simulink model "engine_with_transmission"  (R2026a)
settings: Solver=VariableStepAuto  StopTime=10
libraries: fl_lib x45, nesl_utility x29, sdl_lib x14
settings Model: Creator=doyeop  LastModifiedBy=doyeop

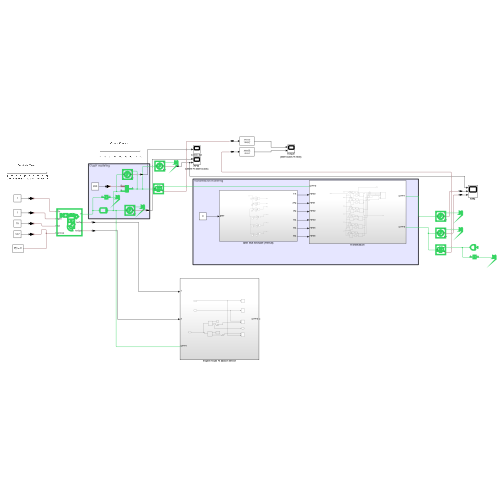
[thumbnail: Simulink's stored preview of the top-level diagram]
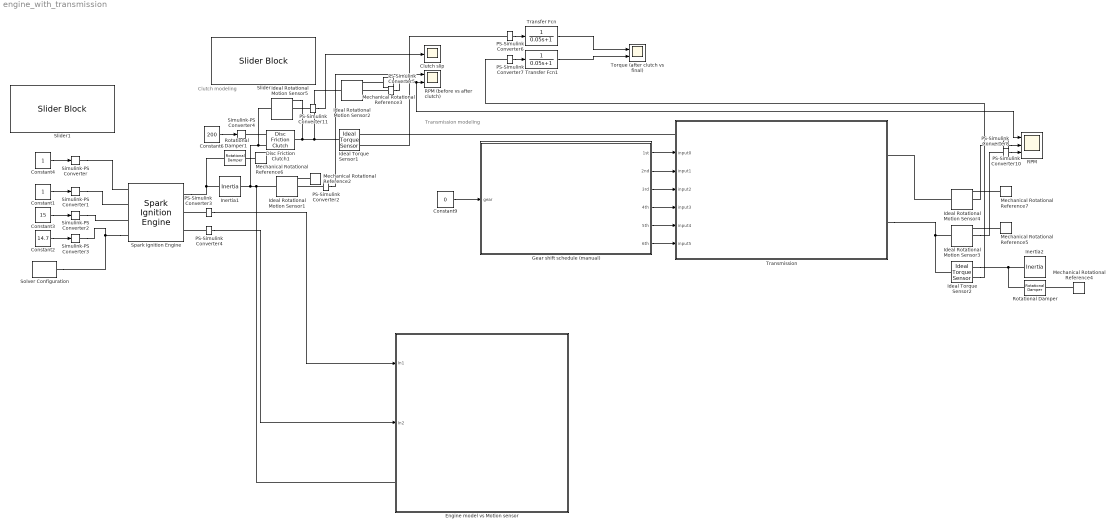
== system engine_with_transmission ==
  note: Transmission modeling
  note: Clutch modeling
  Clutch slip : Scope
      settings: ActiveDisplayYMinimum=-1  ActiveDisplayYMaximum=1  DataLoggingVariableName=ScopeData8
  Constant1 : Constant
  Constant2 : Constant  Value=14.7  SampleTime=-1
  Constant3 : Constant  Value=15  SampleTime=-1
  Constant4 : Constant  SampleTime=-1
  Constant6 : Constant  Value=200  SampleTime=-1
  Constant9 : Constant  Value=0
  Disc Friction Clutch1 : sdl_lib/Clutches/Disc Friction Clutch  geometry_model=sdl.enum.friction_geometry.radius  r_eff=130 mm  d_o=150 mm  d_i=100 mm  nS=4  piston_area=0.001 m^2  unidirectional=sdl.enum.directionality.bidirectional  friction_model=sdl.enum.friction_model_TLU_thermal.fixed  mu_w_vector=[0, 100, 1000] rad/s  temperature_TLU=[280, 300, 320] K  mu_static=0.35  mu_static_vector=[.4, .38, .36]  mu_coulomb=0.3  mu_coulomb_vector=[.3, .22, .19]  mu_coulomb_temp_vector=[.3, .28, .25]  mu_coulomb_matrix=[.34, .32, .3; .3, .28, .25; .25, .2, .15]  mu_interp_method=simscape.enum.interpolation.linear  mu_extrap_method=simscape.enum.extrapolation.linear  d_f=1  w_tol=0.001 rad/s  pressure_min=100 Pa  mu_visc=0 N*m*s/rad  initial_state_locked=sdl.enum.initial_lock.unlocked  thermal_mass=50 kJ/K  T_init=300 K
  Engine model vs Motion sensor : Subsystem
  Gear shift schedule (manual) : Subsystem
  Ideal Rotational Motion Sensor{1..5} (5 alike) : fl_lib/Mechanical/Mechanical Sensors/Ideal Rotational Motion Sensor  reference=foundation.enum.MeasurementReference.difference  acceleration_port=false  velocity_port=true  position_port=true  wrap_angle=false  offset=0 rad
  Ideal Torque Sensor1 : fl_lib/Mechanical/Mechanical Sensors/Ideal Torque Sensor
  Ideal Torque Sensor2 : fl_lib/Mechanical/Mechanical Sensors/Ideal Torque Sensor
  Inertia1 : fl_lib/Mechanical/Rotational Elements/Inertia  inertia=0.01 kg*m^2  num_ports=foundation.enum.numPorts2.two  w_specify=on  w_priority=Low  w=800 rpm  w_nominal_specify=off  w_nominal_value=1  w_nominal_unit=rad/s  t_specify=off  t_priority=None  t=0 N*m  t_nominal_specify=off  t_nominal_value=1  t_nominal_unit=N*m
  Inertia2 : fl_lib/Mechanical/Rotational Elements/Inertia  inertia=0.05 kg*m^2  num_ports=foundation.enum.numPorts2.one  w_specify=on  w_priority=None  w=0 rpm  w_nominal_specify=off  w_nominal_value=1  w_nominal_unit=rad/s  t_specify=off  t_priority=None  t=0 N*m  t_nominal_specify=off  t_nominal_value=1  t_nominal_unit=N*m
  Mechanical Rotational Reference{2..7} (6 alike) : fl_lib/Mechanical/Rotational Elements/Mechanical Rotational Reference
  PS-Simulink Converter{2,4..5,8,10..11} (6 alike) : nesl_utility/PS-Simulink Converter  PhysicalDomain=network_engine_domain  SubClassName=ps_output  LeftPortType=input  RightPortType=output  PseudoPeriodic=off  Frequencies=[]  VectorFormat=inherit  Unit=rpm  AffineConversion=off
  PS-Simulink Converter3 : nesl_utility/PS-Simulink Converter  PhysicalDomain=network_engine_domain  SubClassName=ps_output  LeftPortType=input  RightPortType=output  PseudoPeriodic=off  Frequencies=[]  VectorFormat=inherit  Unit=N*m  AffineConversion=off
  PS-Simulink Converter6 : nesl_utility/PS-Simulink Converter  PhysicalDomain=network_engine_domain  SubClassName=ps_output  LeftPortType=input  RightPortType=output  PseudoPeriodic=off  Frequencies=[]  VectorFormat=inherit  Unit=N*m  AffineConversion=off
  PS-Simulink Converter7 : nesl_utility/PS-Simulink Converter  PhysicalDomain=network_engine_domain  SubClassName=ps_output  LeftPortType=input  RightPortType=output  PseudoPeriodic=off  Frequencies=[]  VectorFormat=inherit  Unit=N*m  AffineConversion=off
  RPM : Scope  NumInputPorts=3
      settings: ActiveDisplayYMinimum=-660.08766248050983  ActiveDisplayYMaximum=5940.7889623245892  DataLoggingVariableName=ScopeData3
  RPM (before vs after clutch) : Scope  NumInputPorts=2
      settings: ActiveDisplayYMinimum=-469.45450664319611  ActiveDisplayYMaximum=4225.0905597887659  DataLoggingVariableName=ScopeData2
  Rotational Damper : fl_lib/Mechanical/Rotational Elements/Rotational Damper  D=0.05 N*m*s/rad  w_specify=off  w_priority=None  w=0 rad/s  w_nominal_specify=off  w_nominal_value=1  w_nominal_unit=rad/s  t_specify=off  t_priority=None  t=0 N*m  t_nominal_specify=off  t_nominal_value=1  t_nominal_unit=N*m
  Rotational Damper1 : fl_lib/Mechanical/Rotational Elements/Rotational Damper  D=0.05 N*m*s/rad  w_specify=off  w_priority=None  w=0 rad/s  w_nominal_specify=off  w_nominal_value=1  w_nominal_unit=rad/s  t_specify=off  t_priority=None  t=0 N*m  t_nominal_specify=off  t_nominal_value=1  t_nominal_unit=N*m
  Simulink-PS Converter : nesl_utility/Simulink-PS Converter  PhysicalDomain=network_engine_domain  SubClassName=ps_input  LeftPortType=input  RightPortType=output  PseudoPeriodic=off  Frequencies=[]  NoiseDistribution=none  NoiseParameters=[]  Unit=1  AffineConversion=off  FilteringAndDerivatives=provide  SimscapeFilterOrder=1  InputFilterTimeConstant=0.001  UdotUserProvided=0
  Simulink-PS Converter1 : nesl_utility/Simulink-PS Converter  PhysicalDomain=network_engine_domain  SubClassName=ps_input  LeftPortType=input  RightPortType=output  PseudoPeriodic=off  Frequencies=[]  NoiseDistribution=none  NoiseParameters=[]  Unit=1  AffineConversion=off  FilteringAndDerivatives=provide  SimscapeFilterOrder=1  InputFilterTimeConstant=0.001  UdotUserProvided=0
  Simulink-PS Converter2 : nesl_utility/Simulink-PS Converter  PhysicalDomain=network_engine_domain  SubClassName=ps_input  LeftPortType=input  RightPortType=output  PseudoPeriodic=off  Frequencies=[]  NoiseDistribution=none  NoiseParameters=[]  Unit=deg  AffineConversion=off  FilteringAndDerivatives=provide  SimscapeFilterOrder=1  InputFilterTimeConstant=0.001  UdotUserProvided=0
  Simulink-PS Converter3 : nesl_utility/Simulink-PS Converter  PhysicalDomain=network_engine_domain  SubClassName=ps_input  LeftPortType=input  RightPortType=output  PseudoPeriodic=off  Frequencies=[]  NoiseDistribution=none  NoiseParameters=[]  Unit=1  AffineConversion=off  FilteringAndDerivatives=provide  SimscapeFilterOrder=1  InputFilterTimeConstant=0.001  UdotUserProvided=0
  Simulink-PS Converter4 : nesl_utility/Simulink-PS Converter  PhysicalDomain=network_engine_domain  SubClassName=ps_input  LeftPortType=input  RightPortType=output  PseudoPeriodic=off  Frequencies=[]  NoiseDistribution=none  NoiseParameters=[]  Unit=kPa  AffineConversion=off  FilteringAndDerivatives=provide  SimscapeFilterOrder=1  InputFilterTimeConstant=0.001  UdotUserProvided=0
  Slider : SliderBlock  ScaleMax=200
  Slider1 : SliderBlock  ScaleMax=1
  Solver Configuration : nesl_utility/Solver Configuration  PhysicalDomain=network_engine_domain  SubClassName=solver  LeftPortType=input  RightPortType=generic  Tones=[]  Harmonics=[]  SimulateNoise=off  Profile=off  UseLocalSampling=off  EnableSwitchedLinearOptims=on  FrequencyDomain=off  UseCCode=off  RelTol=0.001  AbsTol=0.001  MinStep=1e-09  ToWorkspace=off  RevertToSquareIcSolve=off  NumHomotopyIterations=100  PhasorMode=off  PhasorModeNumHarmonics=1  ConsistencySolver=NEWTON_XTOL_AFTER_FTOL  CanonicalOrdering=CANONICAL  OptimizeIntermediates=OPTIMIZED  IndexReductionMethod=DerivativeReplacement  DoDC=off  ResidualTolerance=1e-09  ConsistencyTolSource=GLOBAL  ConsistencyAbsTol=0.001  ConsistencyRelTol=0.001  ConsistencyTolFactor=0.001  UseLocalSolver=off  LocalSolverChoice=NE_BACKWARD_EULER_ADVANCER  ResolveIndetEquations=on  FunctionEvalNumThread=1  LocalSolverSampleTime=0.001  DoFixedCost=off  MaxNonlinIter=3  MaxModeIter=2  ComputeImpulses=off  ImpulseIterations=2  LinearAlgebra=auto  LinearAlgebraNumThread=0  EquationFormulation=NE_TIME_EF  DelaysMemoryBudget=1024  AutomaticFiltering=on  FilteringTimeConstant=0.001  PartitionStorageMethod=AS_NEEDED  PartitionMemoryBudget=1024  PartitionMethod=ROBUST  MultibodyUseLocalSolver=off  MultibodyLocalSolverChoice=ODE1  MultibodyLocalSolverSampleTime=0.001
  Spark Ignition Engine : sdl_lib/Engines & Motors/Spark Ignition Engine  numCyls=sdl.enum.engineNumCylinders.Four  twoCylSADiff=270 deg  L4FiringOrder=sdl.enum.engineFiringOrderFourCylinders.L4_1342  bore=67 mm  stroke=42.5 mm  conrod=90 mm  CR=12.2  P_amb=101.325 kPa  T_amb=298.15 K  rho_air=1.225 mg/cm^3  R_air=288.1965 J/(K*kg)  UseAirIntake=true  c_thr=0.1 s  thr_rest=3 deg  D_plate=5 cm  S_leak=1 cm^2  V_im=500 cm^3  Cd_in=0.9  IVO_0=-10 deg  IVC_0=100 deg  EVO_0=30 deg  EVC_0=5 deg  UseInVVT=false  UseExVVT=false  q_LHV=44.3 MJ/kg  InputAFR=true  AFR_const=14.6  InputInjPw=false  Sinj=6.5 mg/ms  SparkInputType=sdl.enum.engineSparkInputType.Angle  SA_const=20 deg  comb_bd=50 deg  dt_Pcyl_slow_decay=60 s  dt_Tcyl_slow_decay=600 s  dt_exh_decay=5 ms  InputBackPressure=false  dP_exh=50 kPa  dw_exh=6000 rpm  UseExhaustThermal=true  S_exh=1 m^2  M_exh=5 kg  C_exh=100 J/(K*kg)  k_gas=10 s  h_convection=100 W/(K*m^2)  k_radiation=0.3  SB=5.7e-8 W/(K^4*m^2)  Pim_0=101.325 kPa  ca0=0 deg  w0=800 rpm  EngSpdSimLimit=16000 rpm  OutputTorqueAvr=true  OutputSpeedAvr=true  OutputCrkpos=false  OutputPim=false  OutputAirMassFlow=false  OutputFuelMassFlow=false  OutputAFR=false  OutputVcyl=false  OutputPcyl=false  OutputTcyl=false  OutputTexh=false
  "Torque (after clutch vs final) " : Scope  NumInputPorts=2
      settings: ActiveDisplayYMinimum=-0.0058759515011631959  ActiveDisplayYMaximum=0.05288356351046878  DataLoggingVariableName=ScopeData4
  Transfer Fcn : TransferFcn  Denominator=[0.05 1]
  Transfer Fcn1 : TransferFcn  Denominator=[0.05 1]
  Transmission : Subsystem
      settings: PortSchema="{\"entries\":[{\"content\":{\"sides\":[{\"content\":{\"connectorIds\":[\"LConn1\",\"In1\",\"In2\",\"In3\",\"In4\",\"In5\",\"In6\"]},\"type\":\"ConnectorPlacement.EquallySpacedRectSide\",\"uuid\":\"874bf634-2070-4cab-8096-5723edc56c05\"},{\"content\":{\"connectorIds\":[\"RConn1\",\"RConn2\"],\"side\":\"RIGHT\"},\"type\":\"ConnectorPlacement.EquallySpacedRectSide\",\"uuid\":\"b78b6a2b-fef4-45c2-824f-57bcce978833\"},{\"content\":{\"side\":\"TOP\"},\"type\":\"ConnectorPlacement.EquallySpacedRectSide\",\"uuid\":\"7ba34083-3a12-47a3-85ce-7fd7a7157d20\"}]},\"type\":\"ConnectorPlacement.EquallySpacedConnector\",\"uuid\":\"33b097a4-8c30-48a7-a645-92ac0257cae5\"}],\"packageUris\":[\"http://schema.mathworks.com/mf0/Connector/R2020b\"],\"version\":\"1.0\"}"
  wires:
  Constant2/1 -> Simulink-PS Converter3/1
  Constant3/1 -> Simulink-PS Converter2/1
  Constant4/1 -> Simulink-PS Converter/1
  Constant1/1 -> Simulink-PS Converter1/1
  PS-Simulink Converter2/1 -> RPM (before vs after clutch)/1
  PS-Simulink Converter5/1 -> RPM/1, RPM (before vs after clutch)/2
  PS-Simulink Converter8/1 -> RPM/3
  PS-Simulink Converter6/1 -> Transfer Fcn/1
  Transfer Fcn/1 -> "Torque (after clutch vs final) "/1
  Transfer Fcn1/1 -> "Torque (after clutch vs final) "/2
  PS-Simulink Converter7/1 -> Transfer Fcn1/1
  Constant6/1 -> Simulink-PS Converter4/1
  PS-Simulink Converter10/1 -> RPM/2
  PS-Simulink Converter11/1 -> Clutch slip/1
  Constant9/1 -> Gear shift schedule (manual)/1(gear)
  Gear shift schedule (manual)/1(1st) -> Transmission/1(input0)
  Gear shift schedule (manual)/2(2nd) -> Transmission/2(input1)
  Gear shift schedule (manual)/3(3rd) -> Transmission/3(input2)
  PS-Simulink Converter3/1 -> Engine model vs Motion sensor/1(In1)
  PS-Simulink Converter4/1 -> Engine model vs Motion sensor/2(In2)
  Gear shift schedule (manual)/4(4th) -> Transmission/4(input3)
  Gear shift schedule (manual)/5(5th) -> Transmission/5(input4)
  Gear shift schedule (manual)/6(6th) -> Transmission/6(input5)
  connections:
  Spark Ignition Engine/LConn4 -- Simulink-PS Converter3/RConn1 -- Solver Configuration/RConn1
  Simulink-PS Converter2/RConn1 -- Spark Ignition Engine/LConn3
  Simulink-PS Converter1/RConn1 -- Spark Ignition Engine/LConn2
  PS-Simulink Converter3/LConn1 -- Spark Ignition Engine/RConn2
  Simulink-PS Converter/RConn1 -- Spark Ignition Engine/LConn1
  Inertia1/RConn1 -- Spark Ignition Engine/RConn1 -- Rotational Damper1/LConn1
  PS-Simulink Converter4/LConn1 -- Spark Ignition Engine/RConn3
  PS-Simulink Converter2/LConn1 -- Ideal Rotational Motion Sensor1/RConn2
  PS-Simulink Converter5/LConn1 -- Ideal Rotational Motion Sensor2/RConn2
  Mechanical Rotational Reference2/LConn1 -- Ideal Rotational Motion Sensor1/RConn1
  Mechanical Rotational Reference3/LConn1 -- Ideal Rotational Motion Sensor2/RConn1
  Mechanical Rotational Reference4/LConn1 -- Rotational Damper/RConn1
  Engine model vs Motion sensor/LConn1 -- Ideal Rotational Motion Sensor1/LConn1 -- Ideal Rotational Motion Sensor5/LConn1 -- Disc Friction Clutch1/LConn2 -- Inertia1/LConn1
  Ideal Rotational Motion Sensor3/RConn2 -- PS-Simulink Converter8/LConn1
  Mechanical Rotational Reference5/LConn1 -- Ideal Rotational Motion Sensor3/RConn1
  PS-Simulink Converter6/LConn1 -- Ideal Torque Sensor1/RConn2
  Ideal Torque Sensor2/RConn1 -- Rotational Damper/LConn1 -- Inertia2/LConn1
  Ideal Torque Sensor2/RConn2 -- PS-Simulink Converter7/LConn1
  Mechanical Rotational Reference6/LConn1 -- Rotational Damper1/RConn1
  Disc Friction Clutch1/LConn1 -- Simulink-PS Converter4/RConn1
  Ideal Rotational Motion Sensor2/LConn1 -- Ideal Torque Sensor1/LConn1 -- Ideal Rotational Motion Sensor5/RConn1 -- Disc Friction Clutch1/RConn1
  Mechanical Rotational Reference7/LConn1 -- Ideal Rotational Motion Sensor4/RConn1
  PS-Simulink Converter10/LConn1 -- Ideal Rotational Motion Sensor4/RConn2
  PS-Simulink Converter11/LConn1 -- Ideal Rotational Motion Sensor5/RConn2
  Ideal Torque Sensor2/LConn1 -- Transmission/RConn2 -- Ideal Rotational Motion Sensor3/LConn1
  Ideal Rotational Motion Sensor4/LConn1 -- Transmission/RConn1
  Transmission/LConn1 -- Ideal Torque Sensor1/RConn1

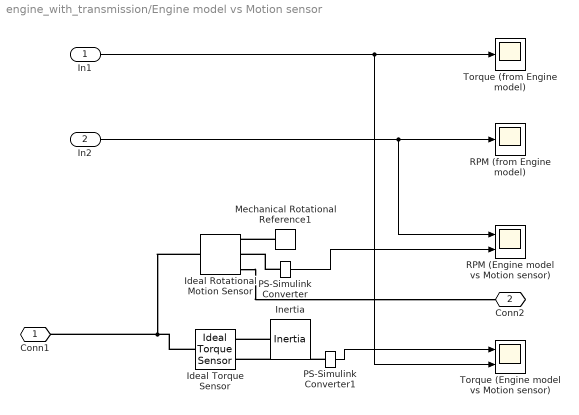
== system engine_with_transmission/Engine model vs Motion sensor ==
  In1 : Inport
  In2 : Inport  Port=2
  Ideal Rotational Motion Sensor : fl_lib/Mechanical/Mechanical Sensors/Ideal Rotational Motion Sensor  reference=foundation.enum.MeasurementReference.difference  acceleration_port=false  velocity_port=true  position_port=true  wrap_angle=false  offset=0 rad
  Ideal Torque Sensor : fl_lib/Mechanical/Mechanical Sensors/Ideal Torque Sensor
  Inertia : fl_lib/Mechanical/Rotational Elements/Inertia  inertia=0.1 kg*m^2  num_ports=foundation.enum.numPorts2.one  w_specify=on  w_priority=None  w=0 rpm  w_nominal_specify=off  w_nominal_value=1  w_nominal_unit=rad/s  t_specify=off  t_priority=None  t=0 N*m  t_nominal_specify=off  t_nominal_value=1  t_nominal_unit=N*m
  Mechanical Rotational Reference1 : fl_lib/Mechanical/Rotational Elements/Mechanical Rotational Reference
  PS-Simulink Converter : nesl_utility/PS-Simulink Converter  PhysicalDomain=network_engine_domain  SubClassName=ps_output  LeftPortType=input  RightPortType=output  PseudoPeriodic=off  Frequencies=[]  VectorFormat=inherit  Unit=rpm  AffineConversion=off
  PS-Simulink Converter1 : nesl_utility/PS-Simulink Converter  PhysicalDomain=network_engine_domain  SubClassName=ps_output  LeftPortType=input  RightPortType=output  PseudoPeriodic=off  Frequencies=[]  VectorFormat=inherit  Unit=N*m  AffineConversion=off
  RPM (Engine model vs Motion sensor) : Scope  NumInputPorts=2
      settings: ActiveDisplayYMinimum=-419.44946675369869  ActiveDisplayYMaximum=3775.0452007832891
  RPM (from Engine model) : Scope
      settings: ActiveDisplayYMinimum=-615.78297464343427  ActiveDisplayYMaximum=5542.04677179091  DataLoggingVariableName=ScopeData6
  Torque (Engine model vs Motion sensor) : Scope  NumInputPorts=2
      settings: ActiveDisplayYMinimum=-41.551396950603035  ActiveDisplayYMaximum=102.79160135138113
  Torque (from Engine model) : Scope
      settings: ActiveDisplayYMinimum=-2.7967171219384035  ActiveDisplayYMaximum=25.170454097445635  DataLoggingVariableName=ScopeData5
  Conn1 : PMIOPort  Side=Left
  Conn2 : PMIOPort  Port=2  Side=Right
  wires:
  PS-Simulink Converter/1 -> RPM (Engine model vs Motion sensor)/2
  In2/1 -> RPM (from Engine model)/1, RPM (Engine model vs Motion sensor)/1
  In1/1 -> Torque (Engine model vs Motion sensor)/2, Torque (from Engine model)/1
  PS-Simulink Converter1/1 -> Torque (Engine model vs Motion sensor)/1
  connections:
  PS-Simulink Converter1/LConn1 -- Ideal Torque Sensor/RConn2
  Mechanical Rotational Reference1/LConn1 -- Ideal Rotational Motion Sensor/RConn1
  PS-Simulink Converter/LConn1 -- Ideal Rotational Motion Sensor/RConn2
  Ideal Torque Sensor/LConn1 -- Ideal Rotational Motion Sensor/LConn1 -- Conn1/RConn1
  Inertia/LConn1 -- Ideal Torque Sensor/RConn1
  Ideal Rotational Motion Sensor/RConn3 -- Conn2/RConn1

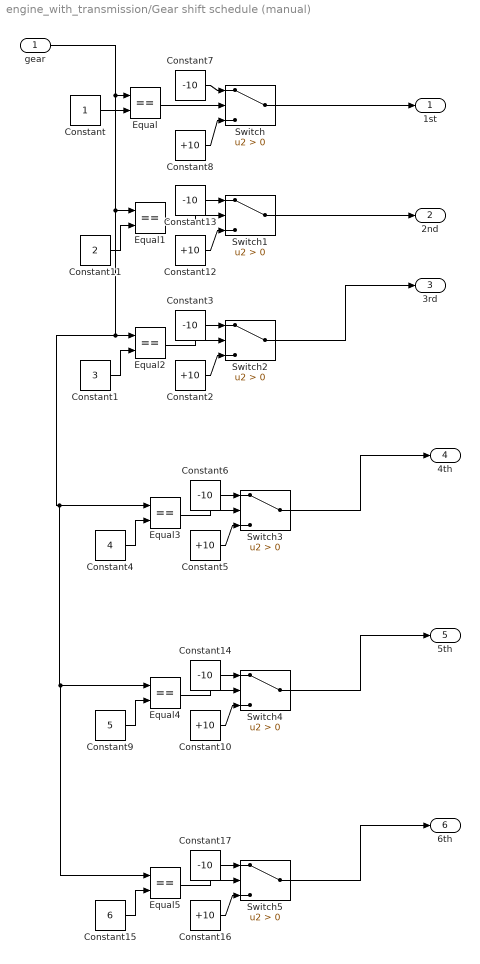
== system engine_with_transmission/Gear shift schedule (manual) ==
  gear : Inport
  Constant : Constant
  Constant1 : Constant  Value=3
  Constant{2,5,8,10,12,16} (6 alike) : Constant  Value=+10  SampleTime=-1
  Constant11 : Constant  Value=2
  Constant{3,6..7,13..14,17} (6 alike) : Constant  Value=-10  SampleTime=-1
  Constant15 : Constant  Value=6
  Constant4 : Constant  Value=4
  Constant9 : Constant  Value=5
  Equal{,1..5} (6 alike) : RelationalOperator  Operator===  OutDataTypeStr=boolean  RndMeth=Simplest  InputSameDT=off
  Switch{,1..5} (6 alike) : Switch  Criteria=u2 > Threshold  SaturateOnIntegerOverflow=off  InputSameDT=off
  1st : Outport
  2nd : Outport  Port=2
  3rd : Outport  Port=3
  4th : Outport  Port=4
  5th : Outport  Port=5
  6th : Outport  Port=6
  wires:
  Constant12/1 -> Switch1/3
  Equal1/1 -> Switch1/2
  Constant7/1 -> Switch/1
  Equal/1 -> Switch/2
  Constant11/1 -> Equal1/2
  Constant8/1 -> Switch/3
  Switch/1 -> 1st/1
  Constant/1 -> Equal/2
  Switch1/1 -> 2nd/1
  Constant13/1 -> Switch1/1
  Constant3/1 -> Switch2/1
  Constant1/1 -> Equal2/2
  Equal2/1 -> Switch2/2
  Constant2/1 -> Switch2/3
  Switch2/1 -> 3rd/1
  Switch3/1 -> 4th/1
  Constant4/1 -> Equal3/2
  Equal3/1 -> Switch3/2
  Constant5/1 -> Switch3/3
  Constant6/1 -> Switch3/1
  Switch4/1 -> 5th/1
  Constant9/1 -> Equal4/2
  Equal4/1 -> Switch4/2
  Constant10/1 -> Switch4/3
  Constant14/1 -> Switch4/1
  Switch5/1 -> 6th/1
  gear/1 -> Equal2/1, Equal5/1, Equal4/1, Equal3/1, Equal1/1, Equal/1
  Constant15/1 -> Equal5/2
  Equal5/1 -> Switch5/2
  Constant16/1 -> Switch5/3
  Constant17/1 -> Switch5/1

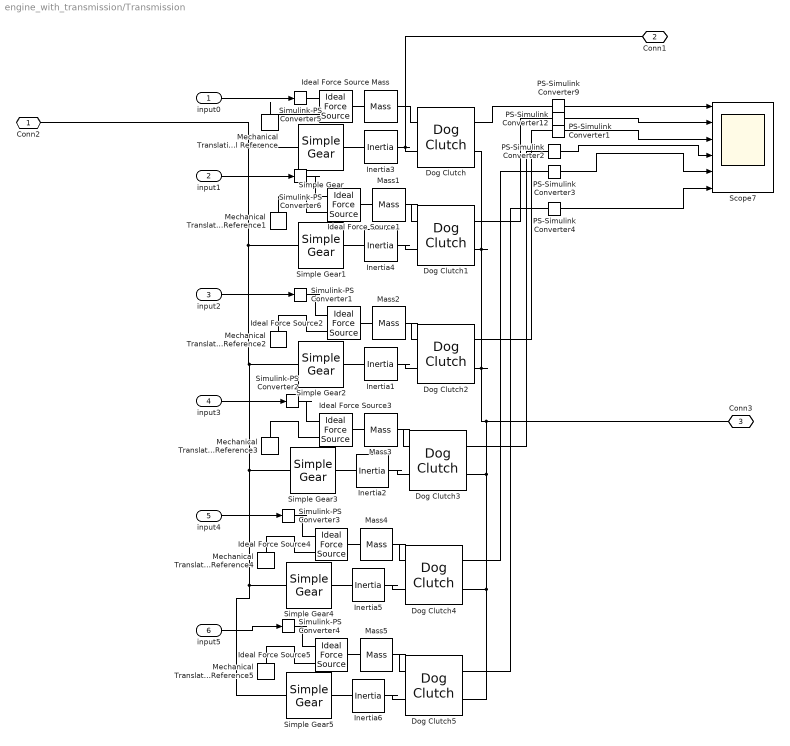
== system engine_with_transmission/Transmission ==
  input0 : Inport
  input1 : Inport  Port=2
  input2 : Inport  Port=3
  input3 : Inport  Port=4
  input4 : Inport  Port=5
  input5 : Inport  Port=6
  Dog Clutch{,1..5} (6 alike) : sdl_lib/Clutches/Dog Clutch  model=sdl.enum.dog_clutch_model.clutch  w_threshold=800 rpm  thermal_port=simscape.enum.thermaleffects.omit  radius=50 mm  max_torque=1000 N*m  n_teeth=6  temperature_TLU=[280, 300, 320] K  max_torque_vector=[1000, 1050, 1000] N*m  interp_method=simscape.enum.interpolation.linear  extrap_method=simscape.enum.extrapolation.linear  clutch_backlash=10 deg  clutch_stiffness=10e6 N*m/rad  clutch_damping=100 N*m*s/rad  shift_linkage_twomode=sdl.enum.shift_linkage_twomode.logic  shift_linkage=sdl.enum.shift_linkage.conserving  tooth_height=10 mm  ring_hub_gap=3 mm  back_stop=true  transl_stiffness=10e5 N/m  transl_damping=1e3 N*s/m  visc_fric_transl=100 N*s/m  engaged_fric_transl=100 N*s/m  disengaged_fric_transl=50 N*s/m  v_tol=0.1 m/s  f_tol=0.001 N  fric_coeff=0.05  direction=sdl.enum.shift_linkage_direction.negative  engagement_velocity=inf rad/s  engagement_overlap=3 mm  engagement_block_stiffness=10e6 N/m  engagement_block_damping=300 N*s/m  initial_state_engaged=false  init_pos=0 mm  init_rel_angle=0 deg  thermal_mass=50 kJ/K  T_init=300 K
  Ideal Force Source{,1..5} (6 alike) : fl_lib/Mechanical/Mechanical Sources/Ideal Force Source
  Inertia{1..6} (6 alike) : fl_lib/Mechanical/Rotational Elements/Inertia  inertia=0.001 kg*m^2  num_ports=foundation.enum.numPorts2.two  w_specify=on  w_priority=High  w=0 rpm  w_nominal_specify=off  w_nominal_value=1  w_nominal_unit=rad/s  t_specify=off  t_priority=None  t=0 N*m  t_nominal_specify=off  t_nominal_value=1  t_nominal_unit=N*m
  Mass{,1..5} (6 alike) : fl_lib/Mechanical/Translational Elements/Mass  mass=0.5 kg  num_ports=foundation.enum.numPorts2.two  v_specify=off  v_priority=High  v=0 m/s  v_nominal_specify=off  v_nominal_value=1  v_nominal_unit=m/s  f_specify=off  f_priority=None  f=0 N  f_nominal_specify=off  f_nominal_value=1  f_nominal_unit=N
  Mechanical Translational Reference{,1..5} (6 alike) : fl_lib/Mechanical/Translational Elements/Mechanical Translational Reference
  PS-Simulink Converter{1..4,9,12} (6 alike) : nesl_utility/PS-Simulink Converter  PhysicalDomain=network_engine_domain  SubClassName=ps_output  LeftPortType=input  RightPortType=output  PseudoPeriodic=off  Frequencies=[]  VectorFormat=inherit  Unit=inherit  AffineConversion=off
  Scope7 : Scope  NumInputPorts=6
      settings: ActiveDisplayYMinimum=-0.01466780214748929  ActiveDisplayYMaximum=0.0016676344827139446  DataLoggingVariableName=ScopeData7
  Simple Gear : sdl_lib/Gears/Simple Gear  ratio=2.75  rotation_direction=sdl.enum.shaftOutputDirection.same  friction_model=sdl.enum.gear_efficiencies_load.off  T_noload=0.1 N*m  T_nom=5 N*m  efficiency_nom=0.8  efficiency=0.8  temperature_TLU=[280, 300, 320] K  load_TLU=[1, 5, 10] N*m  efficiency_TLU=[.95, .9, .85]  efficiency_TLU2=[.85, .8, .75; .95, .9, .85; .85, .8, .7]  w_thr=0.01 rad/s  pwr_thr=0.001 W  enable_backlash=false  hardstop_model=simscape.enum.hardstop.smooth  backlash_distance=1e-3 mm  r_base=0.1 m  transition=1e-4 mm  backlash_stiffness=1e6 N/m  backlash_damping=1e3 N*s/m  coeff_rest=0.7  v_tol=0.001 m/s  f_tol=0.001 N  tau=0.1 s  mu_visc=[0, 0] N*m*s/rad  thermal_mass=50 J/K  temperature_specify=off  temperature_priority=High  temperature=300 K  temperature_nominal_specify=off  temperature_nominal_value=1  temperature_nominal_unit=K  x_backlash_specify=off  x_backlash_priority=None  x_backlash=0 mm  x_backlash_nominal_specify=off  x_backlash_nominal_value=1  x_backlash_nominal_unit=mm  f_hardstop_specify=off  f_hardstop_priority=None  f_hardstop=0 N  f_hardstop_nominal_specify=off  f_hardstop_nominal_value=1  f_hardstop_nominal_unit=N  v_backlash_specify=off  v_backlash_priority=None  v_backlash=0 m/s  v_backlash_nominal_specify=off  v_backlash_nominal_value=1  v_backlash_nominal_unit=m/s
  Simple Gear1 : sdl_lib/Gears/Simple Gear  ratio=2.0  rotation_direction=sdl.enum.shaftOutputDirection.same  friction_model=sdl.enum.gear_efficiencies_load.off  T_noload=0.1 N*m  T_nom=5 N*m  efficiency_nom=0.8  efficiency=0.8  temperature_TLU=[280, 300, 320] K  load_TLU=[1, 5, 10] N*m  efficiency_TLU=[.95, .9, .85]  efficiency_TLU2=[.85, .8, .75; .95, .9, .85; .85, .8, .7]  w_thr=0.01 rad/s  pwr_thr=0.001 W  enable_backlash=false  hardstop_model=simscape.enum.hardstop.smooth  backlash_distance=1e-3 mm  r_base=0.1 m  transition=1e-4 mm  backlash_stiffness=1e6 N/m  backlash_damping=1e3 N*s/m  coeff_rest=0.7  v_tol=0.001 m/s  f_tol=0.001 N  tau=0.1 s  mu_visc=[0, 0] N*m*s/rad  thermal_mass=50 J/K  temperature_specify=off  temperature_priority=High  temperature=300 K  temperature_nominal_specify=off  temperature_nominal_value=1  temperature_nominal_unit=K  x_backlash_specify=off  x_backlash_priority=None  x_backlash=0 mm  x_backlash_nominal_specify=off  x_backlash_nominal_value=1  x_backlash_nominal_unit=mm  f_hardstop_specify=off  f_hardstop_priority=None  f_hardstop=0 N  f_hardstop_nominal_specify=off  f_hardstop_nominal_value=1  f_hardstop_nominal_unit=N  v_backlash_specify=off  v_backlash_priority=None  v_backlash=0 m/s  v_backlash_nominal_specify=off  v_backlash_nominal_value=1  v_backlash_nominal_unit=m/s
  Simple Gear2 : sdl_lib/Gears/Simple Gear  ratio=1.667  rotation_direction=sdl.enum.shaftOutputDirection.same  friction_model=sdl.enum.gear_efficiencies_load.off  T_noload=0.1 N*m  T_nom=5 N*m  efficiency_nom=0.8  efficiency=0.8  temperature_TLU=[280, 300, 320] K  load_TLU=[1, 5, 10] N*m  efficiency_TLU=[.95, .9, .85]  efficiency_TLU2=[.85, .8, .75; .95, .9, .85; .85, .8, .7]  w_thr=0.01 rad/s  pwr_thr=0.001 W  enable_backlash=false  hardstop_model=simscape.enum.hardstop.smooth  backlash_distance=1e-3 mm  r_base=0.1 m  transition=1e-4 mm  backlash_stiffness=1e6 N/m  backlash_damping=1e3 N*s/m  coeff_rest=0.7  v_tol=0.001 m/s  f_tol=0.001 N  tau=0.1 s  mu_visc=[0, 0] N*m*s/rad  thermal_mass=50 J/K  temperature_specify=off  temperature_priority=High  temperature=300 K  temperature_nominal_specify=off  temperature_nominal_value=1  temperature_nominal_unit=K  x_backlash_specify=off  x_backlash_priority=None  x_backlash=0 mm  x_backlash_nominal_specify=off  x_backlash_nominal_value=1  x_backlash_nominal_unit=mm  f_hardstop_specify=off  f_hardstop_priority=None  f_hardstop=0 N  f_hardstop_nominal_specify=off  f_hardstop_nominal_value=1  f_hardstop_nominal_unit=N  v_backlash_specify=off  v_backlash_priority=None  v_backlash=0 m/s  v_backlash_nominal_specify=off  v_backlash_nominal_value=1  v_backlash_nominal_unit=m/s
  Simple Gear3 : sdl_lib/Gears/Simple Gear  ratio=1.444  rotation_direction=sdl.enum.shaftOutputDirection.same  friction_model=sdl.enum.gear_efficiencies_load.off  T_noload=0.1 N*m  T_nom=5 N*m  efficiency_nom=0.8  efficiency=0.8  temperature_TLU=[280, 300, 320] K  load_TLU=[1, 5, 10] N*m  efficiency_TLU=[.95, .9, .85]  efficiency_TLU2=[.85, .8, .75; .95, .9, .85; .85, .8, .7]  w_thr=0.01 rad/s  pwr_thr=0.001 W  enable_backlash=false  hardstop_model=simscape.enum.hardstop.smooth  backlash_distance=1e-3 mm  r_base=0.1 m  transition=1e-4 mm  backlash_stiffness=1e6 N/m  backlash_damping=1e3 N*s/m  coeff_rest=0.7  v_tol=0.001 m/s  f_tol=0.001 N  tau=0.1 s  mu_visc=[0, 0] N*m*s/rad  thermal_mass=50 J/K  temperature_specify=off  temperature_priority=High  temperature=300 K  temperature_nominal_specify=off  temperature_nominal_value=1  temperature_nominal_unit=K  x_backlash_specify=off  x_backlash_priority=None  x_backlash=0 mm  x_backlash_nominal_specify=off  x_backlash_nominal_value=1  x_backlash_nominal_unit=mm  f_hardstop_specify=off  f_hardstop_priority=None  f_hardstop=0 N  f_hardstop_nominal_specify=off  f_hardstop_nominal_value=1  f_hardstop_nominal_unit=N  v_backlash_specify=off  v_backlash_priority=None  v_backlash=0 m/s  v_backlash_nominal_specify=off  v_backlash_nominal_value=1  v_backlash_nominal_unit=m/s
  Simple Gear4 : sdl_lib/Gears/Simple Gear  ratio=1.304  rotation_direction=sdl.enum.shaftOutputDirection.same  friction_model=sdl.enum.gear_efficiencies_load.off  T_noload=0.1 N*m  T_nom=5 N*m  efficiency_nom=0.8  efficiency=0.8  temperature_TLU=[280, 300, 320] K  load_TLU=[1, 5, 10] N*m  efficiency_TLU=[.95, .9, .85]  efficiency_TLU2=[.85, .8, .75; .95, .9, .85; .85, .8, .7]  w_thr=0.01 rad/s  pwr_thr=0.001 W  enable_backlash=false  hardstop_model=simscape.enum.hardstop.smooth  backlash_distance=1e-3 mm  r_base=0.1 m  transition=1e-4 mm  backlash_stiffness=1e6 N/m  backlash_damping=1e3 N*s/m  coeff_rest=0.7  v_tol=0.001 m/s  f_tol=0.001 N  tau=0.1 s  mu_visc=[0, 0] N*m*s/rad  thermal_mass=50 J/K  temperature_specify=off  temperature_priority=High  temperature=300 K  temperature_nominal_specify=off  temperature_nominal_value=1  temperature_nominal_unit=K  x_backlash_specify=off  x_backlash_priority=None  x_backlash=0 mm  x_backlash_nominal_specify=off  x_backlash_nominal_value=1  x_backlash_nominal_unit=mm  f_hardstop_specify=off  f_hardstop_priority=None  f_hardstop=0 N  f_hardstop_nominal_specify=off  f_hardstop_nominal_value=1  f_hardstop_nominal_unit=N  v_backlash_specify=off  v_backlash_priority=None  v_backlash=0 m/s  v_backlash_nominal_specify=off  v_backlash_nominal_value=1  v_backlash_nominal_unit=m/s
  Simple Gear5 : sdl_lib/Gears/Simple Gear  ratio=1.208  rotation_direction=sdl.enum.shaftOutputDirection.same  friction_model=sdl.enum.gear_efficiencies_load.off  T_noload=0.1 N*m  T_nom=5 N*m  efficiency_nom=0.8  efficiency=0.8  temperature_TLU=[280, 300, 320] K  load_TLU=[1, 5, 10] N*m  efficiency_TLU=[.95, .9, .85]  efficiency_TLU2=[.85, .8, .75; .95, .9, .85; .85, .8, .7]  w_thr=0.01 rad/s  pwr_thr=0.001 W  enable_backlash=false  hardstop_model=simscape.enum.hardstop.smooth  backlash_distance=1e-3 mm  r_base=0.1 m  transition=1e-4 mm  backlash_stiffness=1e6 N/m  backlash_damping=1e3 N*s/m  coeff_rest=0.7  v_tol=0.001 m/s  f_tol=0.001 N  tau=0.1 s  mu_visc=[0, 0] N*m*s/rad  thermal_mass=50 J/K  temperature_specify=off  temperature_priority=High  temperature=300 K  temperature_nominal_specify=off  temperature_nominal_value=1  temperature_nominal_unit=K  x_backlash_specify=off  x_backlash_priority=None  x_backlash=0 mm  x_backlash_nominal_specify=off  x_backlash_nominal_value=1  x_backlash_nominal_unit=mm  f_hardstop_specify=off  f_hardstop_priority=None  f_hardstop=0 N  f_hardstop_nominal_specify=off  f_hardstop_nominal_value=1  f_hardstop_nominal_unit=N  v_backlash_specify=off  v_backlash_priority=None  v_backlash=0 m/s  v_backlash_nominal_specify=off  v_backlash_nominal_value=1  v_backlash_nominal_unit=m/s
  Simulink-PS Converter{1..6} (6 alike) : nesl_utility/Simulink-PS Converter  PhysicalDomain=network_engine_domain  SubClassName=ps_input  LeftPortType=input  RightPortType=output  PseudoPeriodic=off  Frequencies=[]  NoiseDistribution=none  NoiseParameters=[]  Unit=N  AffineConversion=off  FilteringAndDerivatives=provide  SimscapeFilterOrder=1  InputFilterTimeConstant=0.001  UdotUserProvided=0
  Conn2 : PMIOPort  Side=Left
  Conn1 : PMIOPort  Port=2  Side=Right
  Conn3 : PMIOPort  Port=3  Side=Right
  wires:
  input1/1 -> Simulink-PS Converter6/1
  PS-Simulink Converter9/1 -> Scope7/1
  PS-Simulink Converter12/1 -> Scope7/2
  input0/1 -> Simulink-PS Converter5/1
  input2/1 -> Simulink-PS Converter1/1
  PS-Simulink Converter1/1 -> Scope7/3
  input3/1 -> Simulink-PS Converter2/1
  input4/1 -> Simulink-PS Converter3/1
  input5/1 -> Simulink-PS Converter4/1
  PS-Simulink Converter2/1 -> Scope7/4
  PS-Simulink Converter3/1 -> Scope7/5
  PS-Simulink Converter4/1 -> Scope7/6
  connections:
  Simulink-PS Converter6/RConn1 -- Ideal Force Source1/RConn1
  Mass1/LConn1 -- Dog Clutch1/LConn1
  Inertia4/LConn1 -- Dog Clutch1/LConn2
  Mass/RConn1 -- Ideal Force Source/LConn1
  Dog Clutch/LConn2 -- Conn1/RConn1 -- Inertia3/LConn1
  Simple Gear/RConn1 -- Inertia3/RConn1
  PS-Simulink Converter12/LConn1 -- Dog Clutch1/RConn1
  Ideal Force Source1/RConn2 -- Mechanical Translational Reference1/LConn1
  Dog Clutch1/RConn2 -- Dog Clutch2/RConn2 -- Dog Clutch5/RConn2 -- Dog Clutch4/RConn2 -- Dog Clutch3/RConn2 -- Conn3/RConn1 -- Dog Clutch/RConn2
  PS-Simulink Converter9/LConn1 -- Dog Clutch/RConn1
  Mass/LConn1 -- Dog Clutch/LConn1
  Mechanical Translational Reference/LConn1 -- Ideal Force Source/RConn2
  Ideal Force Source1/LConn1 -- Mass1/RConn1
  Simple Gear1/RConn1 -- Inertia4/RConn1
  Simple Gear/LConn1 -- Simple Gear5/LConn1 -- Simple Gear4/LConn1 -- Simple Gear3/LConn1 -- Simple Gear2/LConn1 -- Simple Gear1/LConn1 -- Conn2/RConn1
  Simulink-PS Converter5/RConn1 -- Ideal Force Source/RConn1
  Inertia1/LConn1 -- Dog Clutch2/LConn2
  Mass2/LConn1 -- Dog Clutch2/LConn1
  Ideal Force Source2/LConn1 -- Mass2/RConn1
  Ideal Force Source2/RConn2 -- Mechanical Translational Reference2/LConn1
  Simple Gear2/RConn1 -- Inertia1/RConn1
  Simulink-PS Converter1/RConn1 -- Ideal Force Source2/RConn1
  PS-Simulink Converter1/LConn1 -- Dog Clutch2/RConn1
  Ideal Force Source3/RConn2 -- Mechanical Translational Reference3/LConn1
  Simulink-PS Converter2/RConn1 -- Ideal Force Source3/RConn1
  Mass3/LConn1 -- Dog Clutch3/LConn1
  Inertia2/LConn1 -- Dog Clutch3/LConn2
  Dog Clutch3/RConn1 -- PS-Simulink Converter2/LConn1
  Simple Gear3/RConn1 -- Inertia2/RConn1
  Ideal Force Source3/LConn1 -- Mass3/RConn1
  Ideal Force Source4/RConn2 -- Mechanical Translational Reference4/LConn1
  Simulink-PS Converter3/RConn1 -- Ideal Force Source4/RConn1
  Mass4/LConn1 -- Dog Clutch4/LConn1
  Inertia5/LConn1 -- Dog Clutch4/LConn2
  Dog Clutch4/RConn1 -- PS-Simulink Converter3/LConn1
  Simple Gear4/RConn1 -- Inertia5/RConn1
  Ideal Force Source4/LConn1 -- Mass4/RConn1
  Ideal Force Source5/RConn2 -- Mechanical Translational Reference5/LConn1
  Simulink-PS Converter4/RConn1 -- Ideal Force Source5/RConn1
  Mass5/LConn1 -- Dog Clutch5/LConn1
  Inertia6/LConn1 -- Dog Clutch5/LConn2
  Dog Clutch5/RConn1 -- PS-Simulink Converter4/LConn1
  Simple Gear5/RConn1 -- Inertia6/RConn1
  Ideal Force Source5/LConn1 -- Mass5/RConn1
